simulink model "IP_LQG_Design_Caso2"  (R2024b)
settings: Solver=FixedStepAuto  StartTime=0.0  StopTime=5  FixedStep=0.01  RelTol=1e-3
undefined symbols (not defined in the file): A, B, b, c, C_lqg, g, I, K, kb, kt, l, L, M, m, r, Rm, X0_kalman
libraries: vrlib x3, simulink x3
settings Model: Creator=jitendra  LastModifiedBy=crost
settings DataIOCC: ExternalInput=getinputstruct(op_trim1)  InitialState=getstatestruct(op_trim1)  ReturnWorkspaceOutputs=off
settings DebuggingCC: UnconnectedInputMsg=warning  UnconnectedOutputMsg=warning  UnconnectedLineMsg=warning  ArithmeticOperatorsInVariantConditions=warning
settings ModelReferenceCC: EnableRefExpFcnMdlSchedulingChecks=on
settings SFSimCC: SimUseLocalCustomCode=off  CustomCodeUndefinedFunction=UseInterfaceOnly
settings RTWCC: RTWUseLocalCustomCode=off  GPUComputeCapability=3.5
settings ConfigComp: CovBoundaryAbsTol=1.0e-5

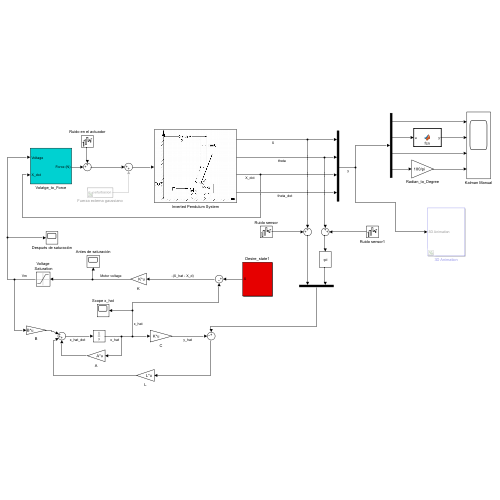
[thumbnail: Simulink's stored preview of the top-level diagram]
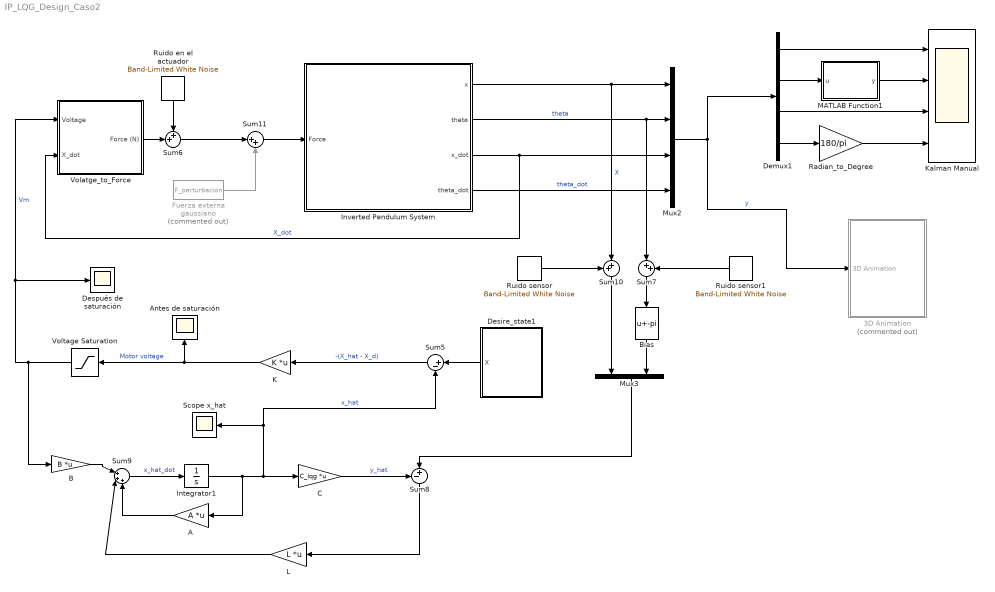
== system IP_LQG_Design_Caso2 ==
  3D Animation : Subsystem  Commented=on
  A : Gain  Gain=A  Multiplication=Matrix(K*u)
  Antes de saturación : Scope
  B : Gain  Gain=B  Multiplication=Matrix(K*u)
  Bias : Bias  Bias=-pi  SaturateOnIntegerOverflow=off
  C : Gain  Gain=C_lqg  Multiplication=Matrix(K*u)
  Demux1 : Demux
  Desire_state1 : Subsystem
  Después de saturación : Scope
  Fuerza externa gaussiano : FromWorkspace  Commented=on  VariableName=F_perturbacion  SampleTime=-1  OutputAfterFinalValue=Setting to zero
  Integrator1 : Integrator  InitialCondition=X0_kalman
  Inverted Pendulum System : Subsystem
      mask Display: image('ip_model.png');
  K : Gain  Gain=K  Multiplication=Matrix(K*u)
  Kalman Manual : Scope  NumInputPorts=4
  L : Gain  Gain=L  Multiplication=Matrix(K*u)
  MATLAB Function1 : MATLAB Function  TreatAsAtomicUnit=on
  Mux2 : Mux
  Mux3 : Mux  Inputs=2
  Radian_to_Degree : Gain  Gain=180/pi
  Ruido en el actuador : simulink/Sources/Band-Limited White Noise  Cov=5.76e-4  Ts=0.01  seed=[23341]
  Ruido sensor : simulink/Sources/Band-Limited White Noise  Cov=6.4e-7  Ts=0.01  seed=[23342]
  Ruido sensor1 : simulink/Sources/Band-Limited White Noise  Cov=1.58e-6  Ts=0.01  seed=[23343]
  Scope x_hat : Scope
  Sum10 : Sum  Inputs=++|
  Sum11 : Sum  Inputs=|++
  Sum5 : Sum  Inputs=|+-
  Sum6 : Sum  Inputs=++|
  Sum7 : Sum  Inputs=|++
  Sum8 : Sum  Inputs=-+|
  Sum9 : Sum  Inputs=|+++
  Volatge_to_Force : Subsystem
  Voltage Saturation : Saturate  UpperLimit=12  LowerLimit=-12
  wires:
  Sum9/1 -> Integrator1/1  "x_hat_dot"
  Fuerza externa gaussiano/1 -> Sum11/2
  Demux1/1 -> Kalman Manual/1
  Sum7/1 -> Bias/1
  Inverted Pendulum System/1(x) -> Sum10/2, Mux2/1  "X"
  K/1 -> Antes de saturación/1, Voltage Saturation/1  "Motor voltage"
  Mux2/1 -> Demux1/1, 3D Animation/1(3D Animation)  "y"
  Integrator1/1 -> A/1, C/1, Scope x_hat/1, Sum5/2  "x_hat"
  Inverted Pendulum System/4(theta_dot) -> Mux2/4  "theta_dot"
  Volatge_to_Force/1(Force (N)) -> Sum6/2
  B/1 -> Sum9/1
  Sum8/1 -> L/1
  Demux1/4 -> Radian_to_Degree/1
  Inverted Pendulum System/3(x_dot) -> Volatge_to_Force/2(X_dot), Mux2/3  "X_dot"
  Inverted Pendulum System/2(theta) -> Mux2/2, Sum7/1  "theta"
  MATLAB Function1/1(y) -> Kalman Manual/2
  L/1 -> Sum9/2
  Demux1/2 -> MATLAB Function1/1(u)
  Ruido en el actuador/1 -> Sum6/1
  C/1 -> Sum8/1  "y_hat"
  Demux1/3 -> Kalman Manual/3
  Voltage Saturation/1 -> B/1, Volatge_to_Force/1(Voltage), Después de saturación/1  "Vm"
  Sum5/1 -> K/1  "-(X_hat - X_d)"
  Ruido sensor/1 -> Sum10/1
  Desire_state1/1(X) -> Sum5/1
  Sum6/1 -> Sum11/1
  Ruido sensor1/1 -> Sum7/2
  Radian_to_Degree/1 -> Kalman Manual/4
  Mux3/1 -> Sum8/2
  Bias/1 -> Mux3/2
  Sum10/1 -> Mux3/1
  A/1 -> Sum9/3
  Sum11/1 -> Inverted Pendulum System/1(Force)

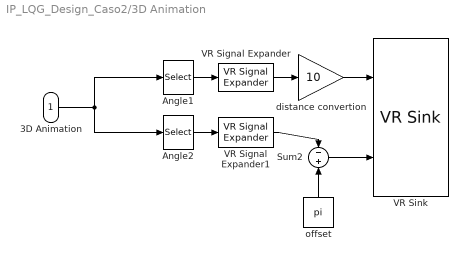
== system IP_LQG_Design_Caso2/3D Animation ==
  3D Animation : Inport
  Angle1 : Selector  InputPortWidth=4  IndexOptions=Index vector (dialog)  Indices=[1]  OutputSizes=1
  Angle2 : Selector  InputPortWidth=4  IndexOptions=Index vector (dialog)  Indices=[2]  OutputSizes=1
  Sum2 : Sum  Inputs=-|+
  VR Signal Expander : vrlib/VR Signal Expander  outwidth=3  outidx=[1]
  VR Signal Expander1 : vrlib/VR Signal Expander  outwidth=4  outidx=[4]
  VR Sink : vrlib/VR Sink  InstantiateOnLoad=on  SampleTime=0.02  ViewEnable=on  RemoteChange=off  RemoteView=off  FieldsWritten=cart.translation.3.1.1.double#joint.rotation.4.1.1.double  WorldFileName=Inverted_pendulum12.wrl  AutoView=off  VideoDimensions=[]  AllowVariableSize=off  FigureProperties=[]
  distance convertion : Gain  Gain=10
  offset : Constant  Value=pi
  wires:
  VR Signal Expander/1 -> distance convertion/1
  3D Animation/1 -> Angle2/1, Angle1/1
  Angle1/1 -> VR Signal Expander/1
  Angle2/1 -> VR Signal Expander1/1
  offset/1 -> Sum2/2
  Sum2/1 -> VR Sink/2
  VR Signal Expander1/1 -> Sum2/1
  distance convertion/1 -> VR Sink/1

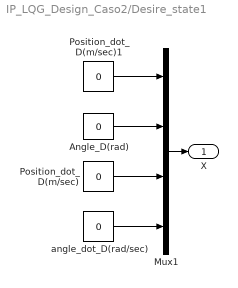
== system IP_LQG_Design_Caso2/Desire_state1 ==
  Angle_D(rad) : Constant  Value=0
  Mux1 : Mux
  Position_dot_D(m/sec) : Constant  Value=0
  Position_dot_D(m/sec)1 : Constant  Value=0
  angle_dot_D(rad/sec) : Constant  Value=0
  X : Outport  VectorParamsAs1DForOutWhenUnconnected=off
  wires:
  Mux1/1 -> X/1
  Position_dot_D(m/sec)/1 -> Mux1/3
  angle_dot_D(rad/sec)/1 -> Mux1/4
  Angle_D(rad)/1 -> Mux1/2
  Position_dot_D(m/sec)1/1 -> Mux1/1

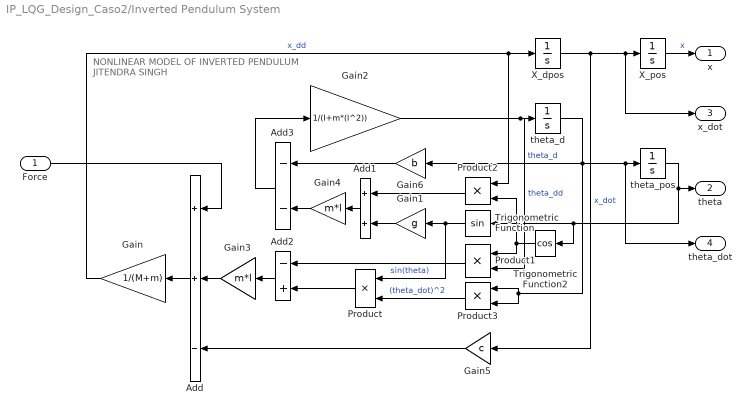
== system IP_LQG_Design_Caso2/Inverted Pendulum System ==
  note: NONLINEAR MODEL OF
      | INVERTED PENDULUM
      | JITENDRA SINGH
  Force : Inport
  Add : Sum  Inputs=++-
  Add1 : Sum
  Add2 : Sum  Inputs=-+
  Add3 : Sum  Inputs=--
  Gain : Gain  Gain=1/(M+m)
  Gain1 : Gain  Gain=g
  Gain2 : Gain  Gain=1/(I+m*(l^2))
  Gain3 : Gain  Gain=m*l
  Gain4 : Gain  Gain=m*l
  Gain5 : Gain  Gain=c
  Gain6 : Gain  Gain=b
  Product{,1..3} (4 alike) : Product
  Trigonometric Function : Trigonometry
  Trigonometric Function2 : Trigonometry  Operator=cos
  X_dpos : Integrator
  X_pos : Integrator  InitialCondition=0.2
  theta_d : Integrator
  theta_pos : Integrator  InitialCondition=160 * (pi/180)
  x : Outport  VectorParamsAs1DForOutWhenUnconnected=off
  theta : Outport  Port=2  VectorParamsAs1DForOutWhenUnconnected=off
  x_dot : Outport  Port=3  VectorParamsAs1DForOutWhenUnconnected=off
  theta_dot : Outport  Port=4  VectorParamsAs1DForOutWhenUnconnected=off
  wires:
  Gain5/1 -> Add/3
  Add2/1 -> Gain3/1
  Add3/1 -> Gain2/1
  Trigonometric Function2/1 -> Product2/2, Product1/1
  Trigonometric Function/1 -> Product/1, Gain1/1  "sin(theta)"
  Gain3/1 -> Add/2
  theta_d/1 -> Product3/2, Product3/1, Gain6/1, theta_dot/1, theta_pos/1  "theta_d"
  Product2/1 -> Add1/1
  Product/1 -> Add2/2
  Gain4/1 -> Add3/2
  Product3/1 -> Product/2  "(theta_dot)^2"
  X_pos/1 -> x/1  "x"
  Product1/1 -> Add2/1
  Gain/1 -> X_dpos/1, Product2/1  "x_dd"
  Add/1 -> Gain/1
  Gain2/1 -> Product1/2, theta_d/1  "theta_dd"
  Gain6/1 -> Add3/1
  theta_pos/1 -> Trigonometric Function2/1, Trigonometric Function/1, theta/1
  Force/1 -> Add/1
  Gain1/1 -> Add1/2
  X_dpos/1 -> x_dot/1, X_pos/1, Gain5/1  "x_dot"
  Add1/1 -> Gain4/1

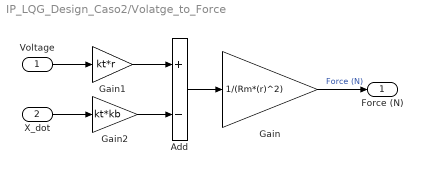
== system IP_LQG_Design_Caso2/Volatge_to_Force ==
  Voltage : Inport
  X_dot : Inport  Port=2
  Add : Sum  Inputs=+-
  Gain : Gain  Gain=1/(Rm*(r)^2)
  Gain1 : Gain  Gain=kt*r
  Gain2 : Gain  Gain=kt*kb
  Force (N) : Outport  VectorParamsAs1DForOutWhenUnconnected=off
  wires:
  Gain1/1 -> Add/1
  Gain2/1 -> Add/2
  Voltage/1 -> Gain1/1
  Gain/1 -> Force (N)/1  "Force (N)"
  X_dot/1 -> Gain2/1
  Add/1 -> Gain/1

== matlab function IP_LQG_Design_Caso2/MATLAB Function1 ==
  data: u input; y output
function y = fcn(u)
    y = mod(u * 180/pi, 360);
end
